simulink model "AnalogIn (1)"  (R2014a)
settings: Solver=FixedStepDiscrete  StartTime=0.0  StopTime=10.0  FixedStep=1  RelTol=1e-3
undefined symbols (not defined in the file): read
libraries: mbed_lib x3
settings Model: Creator=BassAllUser  LastModifiedBy=BassUser
settings OptimizationCC: OptimizeModelRefInitCode=on  LifeSpan=1
settings HardwareCC: ProdBitPerInt=16  ProdBitPerPointer=8  ProdIntDivRoundTo=Zero  ProdEndianess=LittleEndian  ProdWordSize=8  ProdHWDeviceType=Atmel->AVR
settings RTWCC: SystemTargetFile=mbed.tlc  GenCodeOnly=on  PackageGeneratedCodeAndArtifacts=on  PackageName=SimulinkExportPackage  TemplateMakefile=mbed.tmf  Description=mbed  GenerateReport=on  RetainRTWFile=on  ProcessScript=mbed_make_rtw_hook  IncludeHyperlinkInReport=on  LaunchReport=on  TargetLang=C++
settings CodeAppCC: IgnoreCustomStorageClasses=off
settings STFCustomTargetCC: TargetLibSuffix=.a  GenerateSampleERTMain=on  ConcurrentExecutionCompliant=off  GeneratePreprocessorConditionals=Use local settings  CombineOutputUpdateFcns=on  ERTCustomFileBanners=on  SupportContinuousTime=off  SupportNonInlinedSFcns=off  MATLABClassNameForMDSCustomization=Simulink.SoftwareTarget.ERTCustomization  GRTInterface=off  SystemTargetFile=mbed.tlc
settings GRTTargetCC: TargetLibSuffix=.a  GenerateSampleERTMain=on  ParMdlRefBuildCompliant=off  CompOptLevelCompliant=off  ConcurrentExecutionCompliant=off  GeneratePreprocessorConditionals=Use local settings  ERTCustomFileBanners=on  MatFileLogging=off  SupportContinuousTime=off  SupportNonInlinedSFcns=off  MATLABClassNameForMDSCustomization=Simulink.SoftwareTarget.ERTCustomization  CPPClassGenCompliant=off

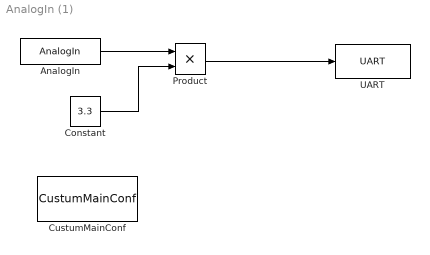
== system AnalogIn (1) ==
  AnalogIn : mbed_lib/AnalogIn  SFunctionSpec=double y1 = dummy(int8 p1,int8 p2, int8 p3)  SParameter1=read()  SParameter2=A0  SParameter3=-1
  Constant : Constant  Value=3.3
  CustumMainConf : mbed_lib/CustumMainConf  P1=main.c  P2=0
  Product : Product
  UART : mbed_lib/UART  SFunctionSpec=double y1 = dummy(int8 p1,int8 p2,int8 p3)  SParameter1=1  SParameter2=ADC Value: read()-> %4.2f Volt\n  SParameter3=-1
  wires:
  AnalogIn/1 -> Product/1
  Constant/1 -> Product/2
  Product/1 -> UART/1
